simulink model "New_model"  (R2021a)
settings: Solver=ode14x  StartTime=0.0  StopTime=100  FixedStep=0.1  RelTol=1e-3
undefined symbols (not defined in the file or in its folder): Ion, Lithium
libraries: fl_lib x29, spsBatteryLib x26, nesl_utility x14, ee_lib x4, sdl_lib x3, spsSeriesRLCLoadLib x2, spsVoltageMeasurementLib x2, spspowerguiLib x2
settings Model: Creator=Zhi Hang  LastModifiedBy=msipc

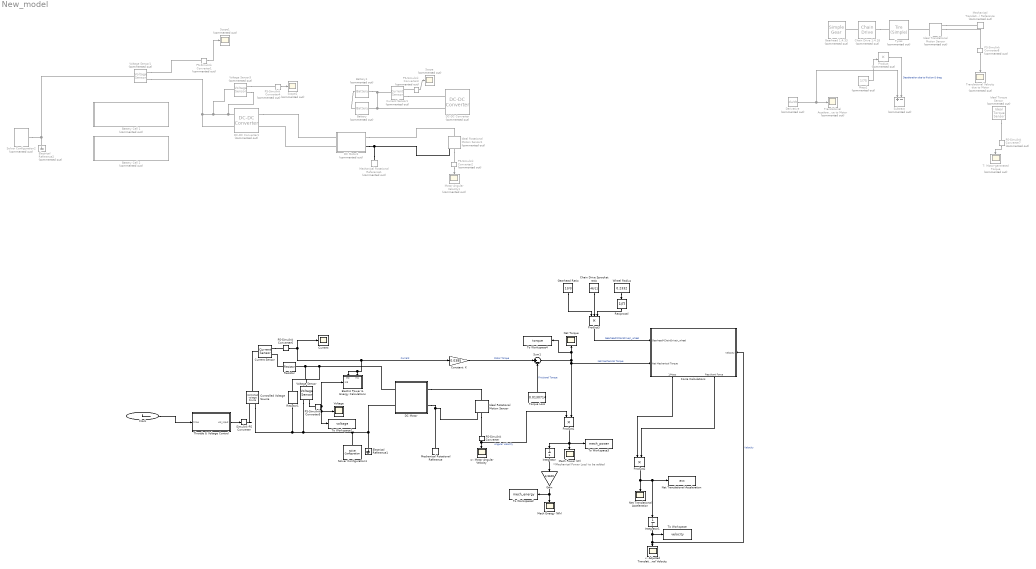
== system New_model ==
  note: *(Mechanical Power Loss) to be added
  Battery : ee_lib/Sources/Battery  Commented=on  Vnom=52 V  prm_dir=1  R1_dis=2 Ohm  R1_ch=2 Ohm  R1=0.26 Ohm  prm_AH=2  AH=2.95 hr*A  V1=45.5 V  AH1=1.385 hr*A  prm_R2=1  R2=2000 Ohm  prm_dyn=1  Rp1=0.005 Ohm  tau1=30 s  Rp2=0.005 Ohm  tau2=30 s  Rp3=0.005 Ohm  tau3=30 s  Rp4=0.005 Ohm  tau4=30 s  Rp5=0.005 Ohm  tau5=30 s  prm_fade=1  N_fade=100  AH_fade=45 hr*A  R1_fade=2.02 Ohm  R1_ch_fade=2.02 Ohm  V1_fade=10.35 V  prm_age=1  prm_age_OCV=1  OCV_age=0.9  SOC_age=60  Tmeas_age=298.15 K  delta_time_age_vec=[0] d  temperature_age_vec=[273] K  OCV_scaling_age=2.2134e6  OCV_offset_age=1.632e6  temp_exp_age=0.515833569 V  t_exp_age=0.75  i_specify=off  i_priority=None  i=0 A  i_nominal_specify=off  i_nominal_unit=A  i_nominal_value=1  v_specify=off  v_priority=None  v=0 V  v_nominal_specify=off  v_nominal_unit=V  v_nominal_value=1  charge_specify=on  charge_priority=High  charge=2.95 hr*A  charge_nominal_specify=off  charge_nominal_unit=hr*A  charge_nominal_value=1  num_cycles_specify=off  num_cycles_priority=High  num_cycles=0  num_cycles_nominal_specify=off  num_cycles_nominal_unit=1  num_cycles_nominal_value=1  thermal_mass=30000 J/K  Tmeas=298.15 K  Vnom_T2=12 V  R1_T2=2.2 Ohm  R1_T2_dis=2.2 Ohm  R1_T2_ch=2.2 Ohm  V1_T2=11.4 V  R2_T2=2200 Ohm  Rp1_T2=0.005 Ohm  tau1_T2=30 s  Rp2_T2=0.005 Ohm  tau2_T2=30 s  Rp3_T2=0.005 Ohm  tau3_T2=30 s  Rp4_T2=0.005 Ohm  tau4_T2=30 s  Rp5_T2=0.005 Ohm  tau5_T2=30 s  Tmeas2=273.15 K  temperature_specify=off  temperature_priority=High  temperature=298.15 K  temperature_nominal_specify=off  temperature_nominal_unit=K  temperature_nominal_value=1
  Battery Cell 1 : Subsystem  Commented=on
  Battery Cell 2 : Subsystem  Commented=on
  Battery1 : ee_lib/Sources/Battery  Commented=on  Vnom=52 V  prm_dir=1  R1_dis=2 Ohm  R1_ch=2 Ohm  R1=0.26 Ohm  prm_AH=2  AH=2.95 hr*A  V1=45.5 V  AH1=1.385 hr*A  prm_R2=1  R2=2000 Ohm  prm_dyn=1  Rp1=0.005 Ohm  tau1=30 s  Rp2=0.005 Ohm  tau2=30 s  Rp3=0.005 Ohm  tau3=30 s  Rp4=0.005 Ohm  tau4=30 s  Rp5=0.005 Ohm  tau5=30 s  prm_fade=1  N_fade=100  AH_fade=45 hr*A  R1_fade=2.02 Ohm  R1_ch_fade=2.02 Ohm  V1_fade=10.35 V  prm_age=1  prm_age_OCV=1  OCV_age=0.9  SOC_age=60  Tmeas_age=298.15 K  delta_time_age_vec=[0] d  temperature_age_vec=[273] K  OCV_scaling_age=2.2134e6  OCV_offset_age=1.632e6  temp_exp_age=0.515833569 V  t_exp_age=0.75  i_specify=off  i_priority=None  i=0 A  i_nominal_specify=off  i_nominal_unit=A  i_nominal_value=1  v_specify=off  v_priority=None  v=0 V  v_nominal_specify=off  v_nominal_unit=V  v_nominal_value=1  charge_specify=on  charge_priority=High  charge=2.95 hr*A  charge_nominal_specify=off  charge_nominal_unit=hr*A  charge_nominal_value=1  num_cycles_specify=off  num_cycles_priority=High  num_cycles=0  num_cycles_nominal_specify=off  num_cycles_nominal_unit=1  num_cycles_nominal_value=1  thermal_mass=30000 J/K  Tmeas=298.15 K  Vnom_T2=12 V  R1_T2=2.2 Ohm  R1_T2_dis=2.2 Ohm  R1_T2_ch=2.2 Ohm  V1_T2=11.4 V  R2_T2=2200 Ohm  Rp1_T2=0.005 Ohm  tau1_T2=30 s  Rp2_T2=0.005 Ohm  tau2_T2=30 s  Rp3_T2=0.005 Ohm  tau3_T2=30 s  Rp4_T2=0.005 Ohm  tau4_T2=30 s  Rp5_T2=0.005 Ohm  tau5_T2=30 s  Tmeas2=273.15 K  temperature_specify=off  temperature_priority=High  temperature=298.15 K  temperature_nominal_specify=off  temperature_nominal_unit=K  temperature_nominal_value=1
  Chain Drive 1:4.18 : sdl_lib/Couplings & Drives/Chain Drive  Commented=on  chain_model=sdl.enum.chain_model.ideal  radius_a=20 mm  radius_b=20*46/11 mm  slack=50 mm  k_chain=1e5 N/m  mu_visc_chain=5 N/(m/s)  mu_visc_a=0 N*m/(rad/s)  mu_visc_b=0 N*m/(rad/s)  breakable=sdl.enum.max_tension.off  F_max=1e6 N  x_specify=off  x_priority=High  x=0 mm  x_nominal_specify=off  x_nominal_unit=mm  x_nominal_value=1
      settings: SourceProductBaseCode=LD  InternalSimscapePortConfiguration="{\"Bottom\":[],\"Left\":[{\"id\":\"A\",\"label\":\"A\",\"type\":\"foundation.mechanical.rotational.rotational\"}],\"Right\":[{\"id\":\"B\",\"label\":\"B\",\"type\":\"foundation.mechanical.rotational.rotational\"}],\"Top\":[]}"
  Chain Drive Sprocket ratio : Constant  Value=46/11
  Clock : Clock
  Constant: K : Gain  Gain=0.0385
  Controlled Voltage Source : fl_lib/Electrical/Electrical Sources/Controlled Voltage Source
  Current : Scope
  Current Sensor : fl_lib/Electrical/Electrical Sensors/Current Sensor
  Current Sensor1 : fl_lib/Electrical/Electrical Sensors/Current Sensor  Commented=on
  DC Motor : Subsystem
  DC Motor1 : Subsystem  Commented=on
  DC-DC Converter : ee_lib/Semiconductors & Converters/Converters/DC-DC Converter  Commented=on  Vref_option=ee.enum.converters.voltageref.internal  v_ref=12 V  P_rated=40 W  droop_param=ee.enum.converters.droop.value  reversible=ee.enum.converters.directionality.unidirectional  losses_option=ee.enum.converters.lossesOption.proportionalToSquaredCurrent  P_fixed=1 W  model_dynamics=ee.enum.converters.dynamics.no  i1_max=15 A  enable_fault=ee.enum.faults.faultEnable.no  fault_condition=ee.enum.faults.faultInputCondition.greaterThan  fault_threshold=0.5  droop=0.8 V/A  droop_percent=2  tau=0.02 s  v_ini=10 V  G_diode=1e-8 1/Ohm  eff_rated=80  i_eff_vec=[1, 2, 3, 4] A  eff_vec=[90, 80, 70, 60]  thermal_mass=100 J/K  initial_temperature=298.15 K  T_eff_vec=[280, 300, 320] K  eff_2D_table=[90, 85, 80; 80, 75, 70; 70, 65, 60; 60, 55, 50]
      settings: SourceProductBaseCode=PS  InternalSimscapePortConfiguration="{\"Bottom\":[],\"Left\":[{\"id\":\"p1\",\"label\":\"1+\",\"type\":\"foundation.electrical.electrical\"},{\"id\":\"n1\",\"label\":\"1-\",\"type\":\"foundation.electrical.electrical\"}],\"Right\":[{\"id\":\"p2\",\"label\":\"2+\",\"type\":\"foundation.electrical.electrical\"},{\"id\":\"n2\",\"label\":\"2-\",\"type\":\"foundation.electrical.electrical\"}],\"Top\":[]}"
  DC-DC Converter1 : ee_lib/Semiconductors & Converters/Converters/DC-DC Converter  Commented=on  Vref_option=ee.enum.converters.voltageref.internal  v_ref=12 V  P_rated=40 W  droop_param=ee.enum.converters.droop.value  reversible=ee.enum.converters.directionality.unidirectional  losses_option=ee.enum.converters.lossesOption.proportionalToSquaredCurrent  P_fixed=1 W  model_dynamics=ee.enum.converters.dynamics.no  i1_max=15 A  enable_fault=ee.enum.faults.faultEnable.no  fault_condition=ee.enum.faults.faultInputCondition.greaterThan  fault_threshold=0.5  droop=0.8 V/A  droop_percent=2  tau=0.02 s  v_ini=10 V  G_diode=1e-8 1/Ohm  eff_rated=91  i_eff_vec=[1, 2, 3, 4] A  eff_vec=[90, 80, 70, 60]  thermal_mass=100 J/K  initial_temperature=298.15 K  T_eff_vec=[280, 300, 320] K  eff_2D_table=[90, 85, 80; 80, 75, 70; 70, 65, 60; 60, 55, 50]
      settings: SourceProductBaseCode=PS  InternalSimscapePortConfiguration="{\"Bottom\":[],\"Left\":[{\"id\":\"p1\",\"label\":\"1+\",\"type\":\"foundation.electrical.electrical\"},{\"id\":\"n1\",\"label\":\"1-\",\"type\":\"foundation.electrical.electrical\"}],\"Right\":[{\"id\":\"p2\",\"label\":\"2+\",\"type\":\"foundation.electrical.electrical\"},{\"id\":\"n2\",\"label\":\"2-\",\"type\":\"foundation.electrical.electrical\"}],\"Top\":[]}"
  Derivative : Derivative  Commented=on
  Electric Power & Energy Calculations : Subsystem
      settings: PortSchema="{\"entries\":[{\"content\":{\"sides\":[{\"content\":{\"connectorIds\":[\"In1\",\"In2\"]},\"type\":\"ConnectorPlacement.EquallySpacedRectSide\",\"uuid\":\"82b9f0de-574e-4e17-acb9-bed6a2542387\"},{\"content\":{\"connectorIds\":[],\"side\":\"RIGHT\"},\"type\":\"ConnectorPlacement.EquallySpacedRectSide\",\"uuid\":\"9cdc9c20-443d-4f74-aa57-a6f03633b23a\"},{\"content\":{\"connectorIds\":[],\"side\":\"TOP\"},\"type\":\"ConnectorPlacement.EquallySpacedRectSide\",\"uuid\":\"5887af2a-3520-4210-9b68-9038b3c81c3d\"},{\"content\":{\"connectorIds\":[\"In3\"],\"side\":\"BOTTOM\"},\"type\":\"ConnectorPlacement.EquallySpacedRectSide\",\"uuid\":\"9e0946f9-9655-43ed-bd46-b30a5293a4ce\"}]},\"type\":\"ConnectorPlacement.EquallySpacedConnector\",\"uuid\":\"9fe55d6d-7bcf-4897-9064-2d765cec3f3f\"}],\"packageUris\":[\"http://schema.mathworks.com/mf0/Connector/R2020b\"],\"version\":\"1.0\"}"
  Electrical Reference1 : fl_lib/Electrical/Electrical Elements/Electrical Reference
  Electrical Reference2 : fl_lib/Electrical/Electrical Elements/Electrical Reference  Commented=on
  Force Calculations : Subsystem
      settings: PortSchema="{\"entries\":[{\"content\":{\"sides\":[{\"content\":{\"connectorIds\":[\"In1\",\"In2\"]},\"type\":\"ConnectorPlacement.EquallySpacedRectSide\",\"uuid\":\"cc3dc385-e02b-45e3-b13c-6583fb37f4e9\"},{\"content\":{\"connectorIds\":[\"In3\"],\"side\":\"RIGHT\"},\"type\":\"ConnectorPlacement.EquallySpacedRectSide\",\"uuid\":\"d2c64c73-4662-4205-87fa-010500d01f5e\"},{\"content\":{\"connectorIds\":[],\"side\":\"TOP\"},\"type\":\"ConnectorPlacement.EquallySpacedRectSide\",\"uuid\":\"e476453e-7c1d-4526-b790-afcebe39b1ff\"},{\"content\":{\"connectorIds\":[\"Out1\",\"Out2\"],\"side\":\"BOTTOM\"},\"type\":\"ConnectorPlacement.EquallySpacedRectSide\",\"uuid\":\"93b3e609-0036-4bd4-a5db-553470fdefa2\"}]},\"type\":\"ConnectorPlacement.EquallySpacedConnector\",\"uuid\":\"e3829ec2-f118-48d6-87d1-cf59a67f9f8c\"}],\"packageUris\":[\"http://schema.mathworks.com/mf0/Connector/R2020b\"],\"version\":\"1.0\"}"
  Gain : Gain  Gain=1/3600
  Gearhead 1:4.33 : sdl_lib/Gears/Simple Gear  Commented=on  ratio=4.33  rotation_direction=sdl.enum.shaftOutputDirection.same  friction_model=sdl.enum.gear_efficiencies_load.constant  mu_visc=[0, 0] N*m/(rad/s)  T_noload=0.1 N*m  T_nom=5 N*m  efficiency_nom=0.8  efficiency=0.9  temperature_TLU=[280, 300, 320] K  load_TLU=[1, 5, 10] N*m  efficiency_TLU=[.95, .9, .85]  efficiency_TLU2=[.85, .8, .75; .95, .9, .85; .85, .8, .7]  w_thr=0.01 rad/s  pwr_thr=0.001 W  thermal_mass=50 J/K  enable_faults=simscape.enum.onoff.off  efficiency_fault=0.05  external_fault=simscape.enum.onoff.off  temporal_fault=simscape.enum.onoff.off  fault_time=5 s  fault_angles=pi / 12 rad  report_fault=simscape.enum.assert.action.none  temperature_specify=off  temperature_priority=High  temperature=300 K  temperature_nominal_specify=off  temperature_nominal_unit=K  temperature_nominal_value=1
  Gearhead Ratio : Constant  Value=13/3
  Ideal Rotational Motion Sensor : fl_lib/Mechanical/Mechanical Sensors/Ideal Rotational Motion Sensor  wrap_angle=simscape.enum.onoff.off  offset=0 rad
  Ideal Rotational Motion Sensor1 : fl_lib/Mechanical/Mechanical Sensors/Ideal Rotational Motion Sensor  Commented=on  wrap_angle=simscape.enum.onoff.off  offset=0 rad
  Ideal Torque Sensor : fl_lib/Mechanical/Mechanical Sensors/Ideal Torque Sensor  Commented=on
  Ideal Translational Motion Sensor : fl_lib/Mechanical/Mechanical Sensors/Ideal Translational Motion Sensor  Commented=on  offset=0 m
  Integrator : Integrator
  Integrator1 : Integrator
  Mass1 : Constant  Commented=on  Value=1/75
  Mech Energy (Wh) : Scope
  Mech Power (W) : Scope
  Mechanical Rotational Reference : fl_lib/Mechanical/Rotational Elements/Mechanical Rotational Reference
  Mechanical Rotational Reference1 : fl_lib/Mechanical/Rotational Elements/Mechanical Rotational Reference  Commented=on
  Mechanical Translational Reference : fl_lib/Mechanical/Translational Elements/Mechanical Translational Reference  Commented=on
  Motor Angular Velocity1 : Scope  Commented=on
  Net Torque : Scope
  Net Translational Acceleration : Scope
  Net Translational Acceleration : ToWorkspace  VariableName=acc  SaveFormat=Timeseries  SampleTime=-1
  PS-Simulink Converter : nesl_utility/PS-Simulink Converter  PhysicalDomain=network_engine_domain  SubClassName=ps_output  LeftPortType=input  RightPortType=output  PseudoPeriodic=off  Frequencies=[]  Unit=inherit  AffineConversion=off
      settings: SourceProductBaseCode=PW,SS
  PS-Simulink Converter{1..4,7..8} (6 alike) : nesl_utility/PS-Simulink Converter  Commented=on  PhysicalDomain=network_engine_domain  SubClassName=ps_output  LeftPortType=input  RightPortType=output  PseudoPeriodic=off  Frequencies=[]  Unit=inherit  AffineConversion=off
      settings: SourceProductBaseCode=PW,SS
  PS-Simulink Converter5 : nesl_utility/PS-Simulink Converter  PhysicalDomain=network_engine_domain  SubClassName=ps_output  LeftPortType=input  RightPortType=output  PseudoPeriodic=off  Frequencies=[]  Unit=inherit  AffineConversion=off
      settings: SourceProductBaseCode=PW,SS
  PS-Simulink Converter6 : nesl_utility/PS-Simulink Converter  PhysicalDomain=network_engine_domain  SubClassName=ps_output  LeftPortType=input  RightPortType=output  PseudoPeriodic=off  Frequencies=[]  Unit=inherit  AffineConversion=off
      settings: SourceProductBaseCode=PW,SS
  Product : Product  Commented=on
  Product1 : Product
  Product2 : Product
  Product3 : Product  Inputs=3
  Reciprocal : Product  Inputs=/
  Resistor : fl_lib/Electrical/Electrical Elements/Resistor  R=1 Ohm  i_specify=off  i_priority=None  i=0 A  i_nominal_specify=off  i_nominal_unit=A  i_nominal_value=1  v_specify=off  v_priority=None  v=0 V  v_nominal_specify=off  v_nominal_unit=V  v_nominal_value=1
  Resistor1 : fl_lib/Electrical/Electrical Elements/Resistor  R=30 Ohm  i_specify=off  i_priority=None  i=0 A  i_nominal_specify=off  i_nominal_unit=A  i_nominal_value=1  v_specify=off  v_priority=None  v=0 V  v_nominal_specify=off  v_nominal_unit=V  v_nominal_value=1
  Scope : Scope  Commented=on
  Scope1 : Scope  Commented=on
  Scope2 : Scope  Commented=on
  Simulink-PS Converter : nesl_utility/Simulink-PS Converter  PhysicalDomain=network_engine_domain  SubClassName=ps_input  LeftPortType=input  RightPortType=output  PseudoPeriodic=off  Frequencies=[]  NoiseDistribution=none  NoiseParameters=[]  Unit=1  AffineConversion=off  FilteringAndDerivatives=filter  SimscapeFilterOrder=1  InputFilterTimeConstant=0.001  UdotUserProvided=0
      settings: SourceProductBaseCode=PW,SS
  Solver Configuration1 : nesl_utility/Solver Configuration  PhysicalDomain=network_engine_domain  SubClassName=solver  LeftPortType=input  RightPortType=generic  Tones=[]  Harmonics=[]  SimulateNoise=off  Profile=off  UseLocalSampling=off  EnableSwitchedLinearOptims=on  FrequencyDomain=off  UseCCode=off  RelTol=0.001  AbsTol=1e-06  MinStep=1e-09  ToWorkspace=off  RevertToSquareIcSolve=off  NumHomotopyIterations=100  PhasorMode=off  PhasorModeNumHarmonics=1  DoDC=off  ResidualTolerance=1e-09  UseLocalSolver=off  LocalSolverChoice=NE_BACKWARD_EULER_ADVANCER  LocalSolverSampleTime=0.001  DoFixedCost=off  MaxNonlinIter=3  MaxModeIter=2  ComputeImpulses=off  ImpulseIterations=2  LinearAlgebra=auto  EquationFormulation=NE_TIME_EF  DelaysMemoryBudget=1024  AutomaticFiltering=on  FilteringTimeConstant=0.001  PartitionStorageMethod=AS_NEEDED  PartitionMemoryBudget=1024  PartitionMethod=ROBUST
      settings: SourceProductBaseCode=PW,SS
  Solver Configuration2 : nesl_utility/Solver Configuration  Commented=on  PhysicalDomain=network_engine_domain  SubClassName=solver  LeftPortType=input  RightPortType=generic  Tones=[]  Harmonics=[]  SimulateNoise=off  Profile=off  UseLocalSampling=off  EnableSwitchedLinearOptims=on  FrequencyDomain=off  UseCCode=off  RelTol=0.001  AbsTol=1e-06  MinStep=1e-09  ToWorkspace=off  RevertToSquareIcSolve=off  NumHomotopyIterations=100  PhasorMode=off  PhasorModeNumHarmonics=1  DoDC=off  ResidualTolerance=1e-09  UseLocalSolver=off  LocalSolverChoice=NE_BACKWARD_EULER_ADVANCER  LocalSolverSampleTime=0.001  DoFixedCost=off  MaxNonlinIter=3  MaxModeIter=2  ComputeImpulses=off  ImpulseIterations=2  LinearAlgebra=auto  EquationFormulation=NE_TIME_EF  DelaysMemoryBudget=1024  AutomaticFiltering=on  FilteringTimeConstant=0.001  PartitionStorageMethod=AS_NEEDED  PartitionMemoryBudget=1024  PartitionMethod=ROBUST
      settings: SourceProductBaseCode=PW,SS
  Subtract : Sum  Commented=on  Inputs=+-
  Sum1 : Sum  Inputs=|+-
  T: Motor-generated Torque : Scope  Commented=on
  Throttle & Voltage Control : MATLAB Function  TreatAsAtomicUnit=on
  To Workspace : ToWorkspace  VariableName=velocity  SaveFormat=Timeseries  SampleTime=-1
  To Workspace1 : ToWorkspace  VariableName=voltage  SaveFormat=Timeseries  SampleTime=-1
  To Workspace2 : ToWorkspace  VariableName=mech_energy  SaveFormat=Timeseries  SampleTime=-1
  To Workspace3 : ToWorkspace  VariableName=mech_power  SaveFormat=Timeseries  SampleTime=-1
  To Workspace4 : ToWorkspace  VariableName=torque  SaveFormat=Timeseries  SampleTime=-1
  Torque Loss : Constant  Value=0.0130714
  Translational Acceleration due to Motor : Scope  Commented=on
  Translational Velocity due to Motor : Scope  Commented=on
  Tyres : sdl_lib/Tires & Vehicles/Tire (Simple)  Commented=on  r_tire=0.2332 m  model_compliance=0  stiffness=1e6 N/m  damping=1000 N/(m/s)  model_inertia=0  tire_inertia=0.5 kg*m^2  initial_velocity=0 rad/s
      settings: SourceProductBaseCode=LD  InternalSimscapePortConfiguration="{\"Bottom\":[],\"Left\":[{\"id\":\"A\",\"label\":\"A\",\"type\":\"foundation.mechanical.rotational.rotational\"}],\"Right\":[{\"id\":\"H\",\"label\":\"H\",\"type\":\"foundation.mechanical.translational.translational\"}],\"Top\":[]}"
  Voltage : Scope
  Voltage Sensor : fl_lib/Electrical/Electrical Sensors/Voltage Sensor
  Voltage Sensor1 : fl_lib/Electrical/Electrical Sensors/Voltage Sensor  Commented=on
  Voltage Sensor3 : fl_lib/Electrical/Electrical Sensors/Voltage Sensor  Commented=on
  Wheel Radius : Constant  Value=0.2332
  v: Adjusted Translational Velocity : Scope
  w: Motor Angular Velocity : Scope
  wires:
  PS-Simulink Converter/1 -> Product1/1, w: Motor Angular Velocity/1  "Angular Velocity"
  PS-Simulink Converter3/1 -> Scope/1
  PS-Simulink Converter1/1 -> Scope1/1
  PS-Simulink Converter2/1 -> Motor Angular Velocity1/1
  PS-Simulink Converter4/1 -> Scope2/1
  PS-Simulink Converter8/1 -> Translational Velocity due to Motor/1
  Derivative/1 -> Subtract/1, Translational Acceleration due to Motor/1
  Mass1/1 -> Product/2
  Clock/1 -> Throttle & Voltage Control/1(time)
  Product/1 -> Subtract/2  "Deceleration due to friction & drag"
  Throttle & Voltage Control/1(vol_input) -> Simulink-PS Converter/1
  Constant: K/1 -> Sum1/1  "Motor Torque"
  PS-Simulink Converter6/1 -> Constant: K/1, Electric Power & Energy Calculations/2(In2), Electric Power & Energy Calculations/1(In1), Current/1  "Current"
  PS-Simulink Converter5/1 -> To Workspace1/1, Voltage/1, Electric Power & Energy Calculations/3(In3)
  PS-Simulink Converter7/1 -> T: Motor-generated Torque/1
  Product2/1 -> Net Translational Acceleration/1, Integrator1/1, Net Translational Acceleration/1
  Integrator1/1 -> v: Adjusted Translational Velocity/1, Force Calculations/3(Velocity), To Workspace/1  "Velocity"
  Sum1/1 -> Product1/2, Force Calculations/2(Net Mechanical Torque), Net Torque/1, To Workspace4/1  "Net Mechanical Torque"
  Torque Loss/1 -> Sum1/2  "Frictional Torque"
  Product1/1 -> Mech Power (W)/1, To Workspace3/1, Integrator/1
  Integrator/1 -> Gain/1
  Wheel Radius/1 -> Reciprocal/1
  Gearhead Ratio/1 -> Product3/1
  Chain Drive Sprocket ratio/1 -> Product3/2
  Reciprocal/1 -> Product3/3
  Gain/1 -> Mech Energy (Wh)/1, To Workspace2/1
  Product3/1 -> Force Calculations/1(Gearhead*ChainDrive/r_wheel)  "Gearhead*ChainDrive/r_wheel"
  Force Calculations/1(1/Mass) -> Product2/1
  Force Calculations/2(Resultant Force) -> Product2/2
  connections:
  DC Motor/RConn1 -- Ideal Rotational Motion Sensor/LConn1
  DC Motor/RConn2 -- Ideal Rotational Motion Sensor/RConn1 -- Mechanical Rotational Reference/LConn1
  Ideal Rotational Motion Sensor/RConn2 -- PS-Simulink Converter/LConn1
  Battery1/RConn1 -- Current Sensor1/LConn1 -- DC-DC Converter/LConn2 -- Battery/RConn1
  Battery/LConn1 -- Battery1/LConn1
  DC Motor/LConn2 -- Controlled Voltage Source/RConn2 -- Resistor1/RConn1 -- Voltage Sensor/RConn2 -- Solver Configuration1/RConn1 -- Electrical Reference1/LConn1
  Current Sensor1/RConn2 -- DC-DC Converter/LConn1
  PS-Simulink Converter3/LConn1 -- Current Sensor1/RConn1
  Solver Configuration2/RConn1 -- Electrical Reference2/LConn1 -- Voltage Sensor1/LConn1
  Voltage Sensor1/RConn1 -- PS-Simulink Converter1/LConn1
  Mechanical Rotational Reference1/LConn1 -- Ideal Rotational Motion Sensor1/RConn1 -- DC Motor1/RConn2
  DC Motor1/RConn1 -- Ideal Rotational Motion Sensor1/LConn1
  Ideal Rotational Motion Sensor1/RConn2 -- PS-Simulink Converter2/LConn1
  DC-DC Converter1/RConn1 -- DC Motor1/LConn1
  DC Motor1/LConn2 -- DC-DC Converter1/RConn2
  Voltage Sensor1/RConn2 -- Voltage Sensor3/LConn1 -- Voltage Sensor3/RConn2 -- DC-DC Converter1/LConn1 -- DC-DC Converter1/LConn2
  Voltage Sensor3/RConn1 -- PS-Simulink Converter4/LConn1
  Chain Drive 1:4.18/LConn1 -- Gearhead 1:4.33/RConn1
  Voltage Sensor/RConn1 -- PS-Simulink Converter5/LConn1
  Chain Drive 1:4.18/RConn1 -- Tyres/LConn1
  Ideal Translational Motion Sensor/LConn1 -- Tyres/RConn1
  Ideal Translational Motion Sensor/RConn1 -- Mechanical Translational Reference/LConn1
  Ideal Translational Motion Sensor/RConn2 -- PS-Simulink Converter8/LConn1
  Simulink-PS Converter/RConn1 -- Controlled Voltage Source/RConn1
  DC Motor/LConn1 -- Voltage Sensor/LConn1 -- Resistor1/LConn1 -- Resistor/RConn1
  Current Sensor/RConn1 -- PS-Simulink Converter6/LConn1
  Ideal Torque Sensor/RConn2 -- PS-Simulink Converter7/LConn1
  Current Sensor/LConn1 -- Controlled Voltage Source/LConn1
  Resistor/LConn1 -- Current Sensor/RConn2

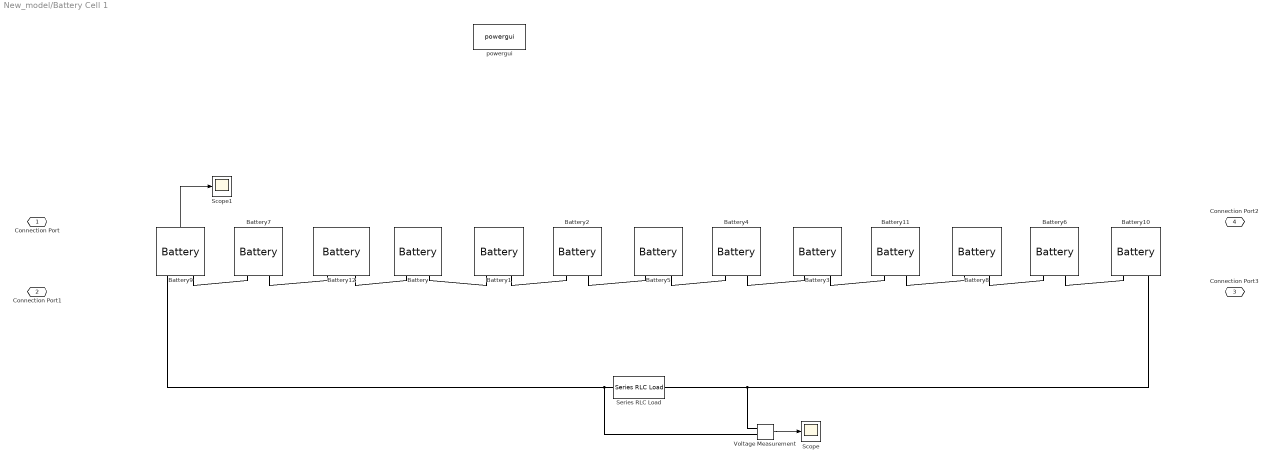
== system New_model/Battery Cell 1 ==
  Battery{,1..12} (13 alike) : spsBatteryLib/Battery  BatType=Lithium-Ion  ShowTempParam=off  ThermalPreset=no  ShowAgeParam=off  NomV=3.61  NomQ=2.95  SOC=100  Batt_Tr=1  PresetModel=off  MaxQ=2.95  MinV=2.5  FullV=4.1  Dis_rate=5  R=0.03  Normal_OP=1.65  expZone=[3.95 0.1]  current=[0 1 2 3 4 5]  Units=Time  Tci=20  NomT=20  T2=-30  MaxQ2=4.8  FullV2=7.1  Normal_OP2=5.655  expZone2="[6.58           1]"  Rca=0.6  ti=2000  Dp=0  Neq0=0  Tsim=1e6  Ta1=25  Qeol=5.4*0.9  Reol=0.013333*1.2  Char_age=[2.3478, 3]  Dis_age=[2.3478, 10]  N1=1500  N2=10500  N3=1000  N4=1400  Ta2=45  N5=950
  Scope : Scope
  Scope1 : Scope
  Series RLC Load : spsSeriesRLCLoadLib/Series RLC Load  LConnTagsString=a  RConnTagsString=__new0  NominalVoltage=1000  NominalFrequency=60  ActivePower=10e4  InductivePower=0  CapacitivePower=0  Setx0=off  InitialVoltage=0  SetiL0=off  InitialCurrent=0  Measurements=None  LoadType=constant Z
  Voltage Measurement : spsVoltageMeasurementLib/Voltage Measurement  PhasorSimulation=off  OutputType=Complex  PSBequivalent=0
  powergui : spspowerguiLib/powergui  Priority=1  SimulationMode=Continuous  SampleTime=50e-6  frequency=60  Iterations=50  frequencyindice=0  Pbase=100e6  ErrMax=1e-4  UnitsV=kV  UnitsW=MW  buscounter=0  FunctionMessages=off  echomessages=off  EnableUseOfTLC=off  CurrentSourceSwitches=off  DisableSnubberDevices=off  DisableRonSwitches=off  DisableVfSwitches=off  DisplayEquations=off  AutomaticDiscreteSolvers=off  SolverType=Tustin/Backward Euler (TBE)  Interpol=off  ExternalGateDelay=off  methode=off  Ts=100  x0status=blocks  SPID=on  SwTol=0  HookPort=off  NonlinearTolerance=1e-4  nMaxIteration=100  ContinueOnMaxIteration=off  RestoreLinks=warning  ResistiveCurrentMeasurement=off  Frange=[0:2:500]  Ylog=off  Xlog=on  ShowGrid=off  save=off  variable=ZData  structure=0  ZoomFFT=off  StartTime=0.0  cycles=1  DisplayStyle=1  fundamental=60  FreqAxis=off  MaxFrequency=1000  frequencyindicesteady=1  RmsSteady=1  display=off
  Connection Port : PMIOPort  Side=Left
  Connection Port1 : PMIOPort  Port=2  Side=Left
  Connection Port3 : PMIOPort  Port=3  Side=Right
  Connection Port2 : PMIOPort  Port=4  Side=Right
  wires:
  Voltage Measurement/1 -> Scope/1
  Battery9/1 -> Scope1/1
  connections:
  Battery9/LConn1 -- Battery7/LConn2
  Battery7/LConn1 -- Battery12/LConn2
  Battery12/LConn1 -- Battery/LConn2
  Battery1/LConn2 -- Battery/LConn1
  Battery1/LConn1 -- Battery2/LConn2
  Battery2/LConn1 -- Battery5/LConn2
  Battery5/LConn1 -- Battery4/LConn2
  Battery4/LConn1 -- Battery3/LConn2
  Battery3/LConn1 -- Battery11/LConn2
  Battery11/LConn1 -- Battery8/LConn2
  Battery8/LConn1 -- Battery6/LConn2
  Battery6/LConn1 -- Battery10/LConn2
  Battery9/LConn2 -- Voltage Measurement/LConn2 -- Series RLC Load/LConn1
  Battery10/LConn1 -- Voltage Measurement/LConn1 -- Series RLC Load/RConn1

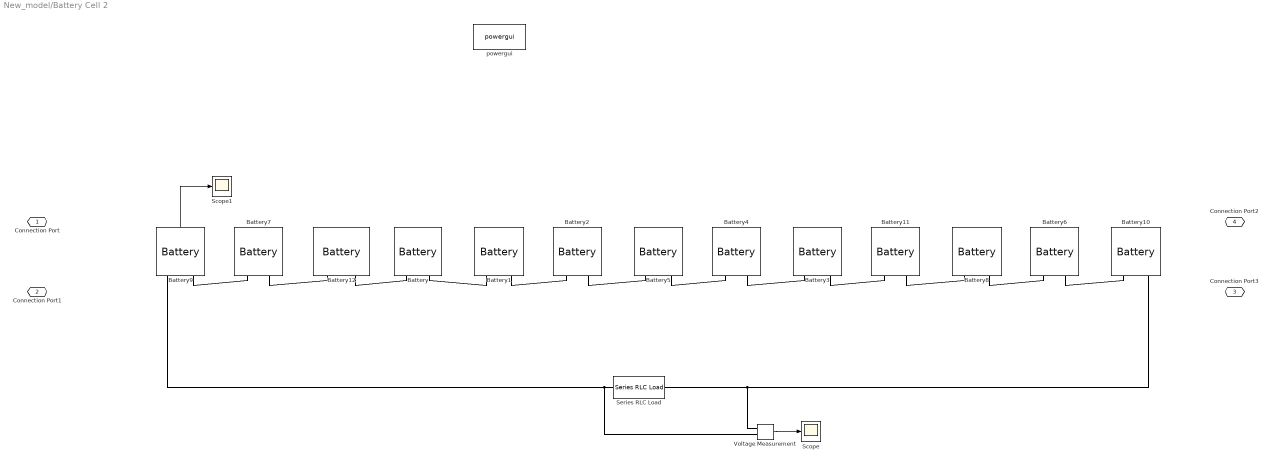
== system New_model/Battery Cell 2 ==
  Battery{,1..12} (13 alike) : spsBatteryLib/Battery  BatType=Lithium-Ion  ShowTempParam=off  ThermalPreset=no  ShowAgeParam=off  NomV=3.61  NomQ=2.95  SOC=100  Batt_Tr=1  PresetModel=off  MaxQ=2.95  MinV=2.5  FullV=4.1  Dis_rate=5  R=0.03  Normal_OP=1.65  expZone=[3.95 0.1]  current=[0 1 2 3 4 5]  Units=Time  Tci=20  NomT=20  T2=-30  MaxQ2=4.8  FullV2=7.1  Normal_OP2=5.655  expZone2="[6.58           1]"  Rca=0.6  ti=2000  Dp=0  Neq0=0  Tsim=1e6  Ta1=25  Qeol=5.4*0.9  Reol=0.013333*1.2  Char_age=[2.3478, 3]  Dis_age=[2.3478, 10]  N1=1500  N2=10500  N3=1000  N4=1400  Ta2=45  N5=950
  Scope : Scope
  Scope1 : Scope
  Series RLC Load : spsSeriesRLCLoadLib/Series RLC Load  LConnTagsString=a  RConnTagsString=__new0  NominalVoltage=1000  NominalFrequency=60  ActivePower=10e4  InductivePower=0  CapacitivePower=0  Setx0=off  InitialVoltage=0  SetiL0=off  InitialCurrent=0  Measurements=None  LoadType=constant Z
  Voltage Measurement : spsVoltageMeasurementLib/Voltage Measurement  PhasorSimulation=off  OutputType=Complex  PSBequivalent=0
  powergui : spspowerguiLib/powergui  Priority=1  SimulationMode=Continuous  SampleTime=50e-6  frequency=60  Iterations=50  frequencyindice=0  Pbase=100e6  ErrMax=1e-4  UnitsV=kV  UnitsW=MW  buscounter=0  FunctionMessages=off  echomessages=off  EnableUseOfTLC=off  CurrentSourceSwitches=off  DisableSnubberDevices=off  DisableRonSwitches=off  DisableVfSwitches=off  DisplayEquations=off  AutomaticDiscreteSolvers=off  SolverType=Tustin/Backward Euler (TBE)  Interpol=off  ExternalGateDelay=off  methode=off  Ts=100  x0status=blocks  SPID=on  SwTol=0  HookPort=off  NonlinearTolerance=1e-4  nMaxIteration=100  ContinueOnMaxIteration=off  RestoreLinks=warning  ResistiveCurrentMeasurement=off  Frange=[0:2:500]  Ylog=off  Xlog=on  ShowGrid=off  save=off  variable=ZData  structure=0  ZoomFFT=off  StartTime=0.0  cycles=1  DisplayStyle=1  fundamental=60  FreqAxis=off  MaxFrequency=1000  frequencyindicesteady=1  RmsSteady=1  display=off
  Connection Port : PMIOPort  Side=Left
  Connection Port1 : PMIOPort  Port=2  Side=Left
  Connection Port3 : PMIOPort  Port=3  Side=Right
  Connection Port2 : PMIOPort  Port=4  Side=Right
  wires:
  Voltage Measurement/1 -> Scope/1
  Battery9/1 -> Scope1/1
  connections:
  Battery9/LConn1 -- Battery7/LConn2
  Battery7/LConn1 -- Battery12/LConn2
  Battery12/LConn1 -- Battery/LConn2
  Battery1/LConn2 -- Battery/LConn1
  Battery1/LConn1 -- Battery2/LConn2
  Battery2/LConn1 -- Battery5/LConn2
  Battery5/LConn1 -- Battery4/LConn2
  Battery4/LConn1 -- Battery3/LConn2
  Battery3/LConn1 -- Battery11/LConn2
  Battery11/LConn1 -- Battery8/LConn2
  Battery8/LConn1 -- Battery6/LConn2
  Battery6/LConn1 -- Battery10/LConn2
  Series RLC Load/LConn1 -- Battery9/LConn2 -- Voltage Measurement/LConn2
  Series RLC Load/RConn1 -- Battery10/LConn1 -- Voltage Measurement/LConn1

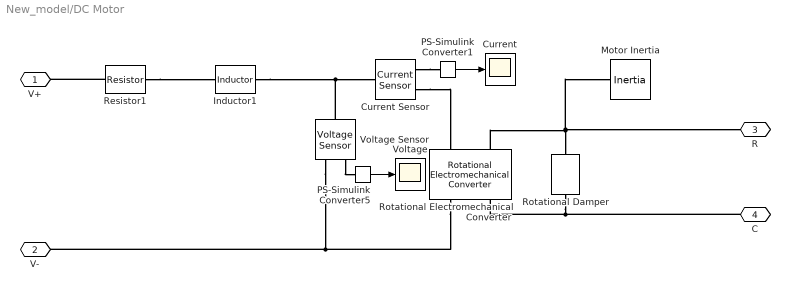
== system New_model/DC Motor ==
  " Motor Inertia" : fl_lib/Mechanical/Rotational Elements/Inertia  inertia=5.48e-5 kg*m^2  num_ports=foundation.enum.numPorts2.one  w_specify=off  w_priority=High  w=0 rad/s  w_nominal_specify=off  w_nominal_unit=rad/s  w_nominal_value=1  t_specify=off  t_priority=None  t=0 N*m  t_nominal_specify=off  t_nominal_unit=N*m  t_nominal_value=1
  Current : Scope
  Current Sensor : fl_lib/Electrical/Electrical Sensors/Current Sensor
  Inductor1 : fl_lib/Electrical/Electrical Elements/Inductor  l=0.072e-3 H  r=0 Ohm  g=1e-9 1/Ohm  i_specify=off  i_priority=None  i=0 A  i_nominal_specify=off  i_nominal_unit=A  i_nominal_value=1  v_specify=off  v_priority=None  v=0 V  v_nominal_specify=off  v_nominal_unit=V  v_nominal_value=1  i_L_specify=off  i_L_priority=High  i_L=0 A  i_L_nominal_specify=off  i_L_nominal_unit=A  i_L_nominal_value=1
  PS-Simulink Converter1 : nesl_utility/PS-Simulink Converter  PhysicalDomain=network_engine_domain  SubClassName=ps_output  LeftPortType=input  RightPortType=output  PseudoPeriodic=off  Frequencies=[]  Unit=inherit  AffineConversion=off
      settings: SourceProductBaseCode=PW,SS
  PS-Simulink Converter5 : nesl_utility/PS-Simulink Converter  PhysicalDomain=network_engine_domain  SubClassName=ps_output  LeftPortType=input  RightPortType=output  PseudoPeriodic=off  Frequencies=[]  Unit=inherit  AffineConversion=off
      settings: SourceProductBaseCode=PW,SS
  Resistor1 : fl_lib/Electrical/Electrical Elements/Resistor  R=0.103 Ohm  i_specify=off  i_priority=None  i=0 A  i_nominal_specify=off  i_nominal_unit=A  i_nominal_value=1  v_specify=off  v_priority=None  v=0 V  v_nominal_specify=off  v_nominal_unit=V  v_nominal_value=1
  Rotational Electromechanical Converter : fl_lib/Electrical/Electrical Elements/Rotational Electromechanical Converter  K=0.0385 V/(rad/s)  i_specify=off  i_priority=None  i=0 A  i_nominal_specify=off  i_nominal_unit=A  i_nominal_value=1  v_specify=off  v_priority=None  v=0 V  v_nominal_specify=off  v_nominal_unit=V  v_nominal_value=1  t_specify=off  t_priority=None  t=0 N*m  t_nominal_specify=off  t_nominal_unit=N*m  t_nominal_value=1  w_specify=off  w_priority=None  w=0 rad/s  w_nominal_specify=off  w_nominal_unit=rad/s  w_nominal_value=1
  Rotational Damper : fl_lib/Mechanical/Rotational Elements/Rotational Damper  D=2.458e-4 N*m/(rad/s)  w_specify=off  w_priority=None  w=0 rad/s  w_nominal_specify=off  w_nominal_unit=rad/s  w_nominal_value=1  t_specify=off  t_priority=None  t=0 N*m  t_nominal_specify=off  t_nominal_unit=N*m  t_nominal_value=1
  Voltage : Scope
  Voltage Sensor : fl_lib/Electrical/Electrical Sensors/Voltage Sensor
  V+ : PMIOPort  Side=Left
  V- : PMIOPort  Port=2  Side=Left
  R : PMIOPort  Port=3  Side=Right
  C : PMIOPort  Port=4  Side=Right
  wires:
  PS-Simulink Converter5/1 -> Voltage/1
  PS-Simulink Converter1/1 -> Current/1
  connections:
  Rotational Electromechanical Converter/LConn2 -- " Motor Inertia"/LConn1 -- R/RConn1 -- Rotational Damper/LConn1
  Resistor1/LConn1 -- V+/RConn1
  Rotational Damper/RConn1 -- C/RConn1 -- Rotational Electromechanical Converter/RConn2
  Rotational Electromechanical Converter/RConn1 -- Voltage Sensor/RConn2 -- V-/RConn1
  Voltage Sensor/RConn1 -- PS-Simulink Converter5/LConn1
  Current Sensor/RConn2 -- Rotational Electromechanical Converter/LConn1
  Current Sensor/RConn1 -- PS-Simulink Converter1/LConn1
  Resistor1/RConn1 -- Inductor1/LConn1
  Inductor1/RConn1 -- Voltage Sensor/LConn1 -- Current Sensor/LConn1

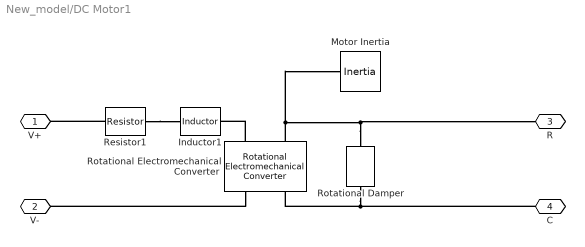
== system New_model/DC Motor1 ==
  " Motor Inertia" : fl_lib/Mechanical/Rotational Elements/Inertia  inertia=0.01 kg*m^2  num_ports=foundation.enum.numPorts2.one  w_specify=off  w_priority=High  w=0 rad/s  w_nominal_specify=off  w_nominal_unit=rad/s  w_nominal_value=1  t_specify=off  t_priority=None  t=0 N*m  t_nominal_specify=off  t_nominal_unit=N*m  t_nominal_value=1
  Inductor1 : fl_lib/Electrical/Electrical Elements/Inductor  l=1e-6 H  r=0 Ohm  g=1e-9 1/Ohm  i_specify=off  i_priority=None  i=0 A  i_nominal_specify=off  i_nominal_unit=A  i_nominal_value=1  v_specify=off  v_priority=None  v=0 V  v_nominal_specify=off  v_nominal_unit=V  v_nominal_value=1  i_L_specify=off  i_L_priority=High  i_L=0 A  i_L_nominal_specify=off  i_L_nominal_unit=A  i_L_nominal_value=1
  Resistor1 : fl_lib/Electrical/Electrical Elements/Resistor  R=1 Ohm  i_specify=off  i_priority=None  i=0 A  i_nominal_specify=off  i_nominal_unit=A  i_nominal_value=1  v_specify=off  v_priority=None  v=0 V  v_nominal_specify=off  v_nominal_unit=V  v_nominal_value=1
  Rotational Electromechanical Converter : fl_lib/Electrical/Electrical Elements/Rotational Electromechanical Converter  K=0.1 V/(rad/s)  i_specify=off  i_priority=None  i=0 A  i_nominal_specify=off  i_nominal_unit=A  i_nominal_value=1  v_specify=off  v_priority=None  v=0 V  v_nominal_specify=off  v_nominal_unit=V  v_nominal_value=1  t_specify=off  t_priority=None  t=0 N*m  t_nominal_specify=off  t_nominal_unit=N*m  t_nominal_value=1  w_specify=off  w_priority=None  w=0 rad/s  w_nominal_specify=off  w_nominal_unit=rad/s  w_nominal_value=1
  Rotational Damper : fl_lib/Mechanical/Rotational Elements/Rotational Damper  D=0.001 N*m/(rad/s)  w_specify=off  w_priority=None  w=0 rad/s  w_nominal_specify=off  w_nominal_unit=rad/s  w_nominal_value=1  t_specify=off  t_priority=None  t=0 N*m  t_nominal_specify=off  t_nominal_unit=N*m  t_nominal_value=1
  V+ : PMIOPort  Side=Left
  V- : PMIOPort  Port=2  Side=Left
  R : PMIOPort  Port=3  Side=Right
  C : PMIOPort  Port=4  Side=Right
  connections:
  Rotational Damper/LConn1 -- " Motor Inertia"/LConn1 -- Rotational Electromechanical Converter/LConn2 -- R/RConn1
  Resistor1/RConn1 -- Inductor1/LConn1
  Resistor1/LConn1 -- V+/RConn1
  Rotational Electromechanical Converter/RConn2 -- Rotational Damper/RConn1 -- C/RConn1
  Rotational Electromechanical Converter/RConn1 -- V-/RConn1
  Rotational Electromechanical Converter/LConn1 -- Inductor1/RConn1

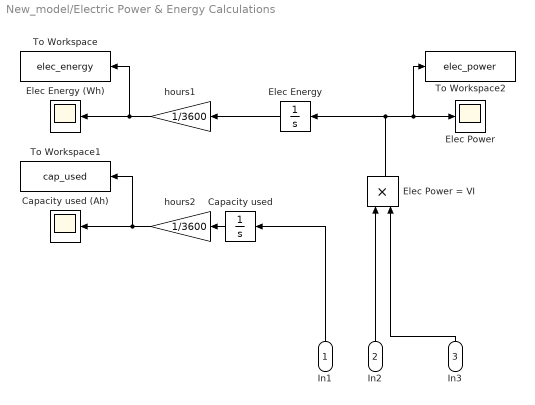
== system New_model/Electric Power & Energy Calculations ==
  In1 : Inport
  In2 : Inport  Port=2
  In3 : Inport  Port=3
  Capacity used : Integrator
  Capacity used (Ah) : Scope
  Elec Energy : Integrator
  Elec Energy (Wh) : Scope
  Elec Power : Scope
  Elec Power = VI : Product
  To Workspace : ToWorkspace  VariableName=elec_energy  SaveFormat=Timeseries  SampleTime=-1
  To Workspace1 : ToWorkspace  VariableName=cap_used  SaveFormat=Timeseries  SampleTime=-1
  To Workspace2 : ToWorkspace  VariableName=elec_power  SaveFormat=Timeseries  SampleTime=-1
  hours1 : Gain  Gain=1/3600
  hours2 : Gain  Gain=1/3600
  wires:
  hours1/1 -> To Workspace/1, Elec Energy (Wh)/1
  In2/1 -> Elec Power = VI/1
  hours2/1 -> Capacity used (Ah)/1, To Workspace1/1
  Elec Power = VI/1 -> Elec Energy/1, To Workspace2/1, Elec Power/1
  In1/1 -> Capacity used/1
  Elec Energy/1 -> hours1/1
  Capacity used/1 -> hours2/1
  In3/1 -> Elec Power = VI/2

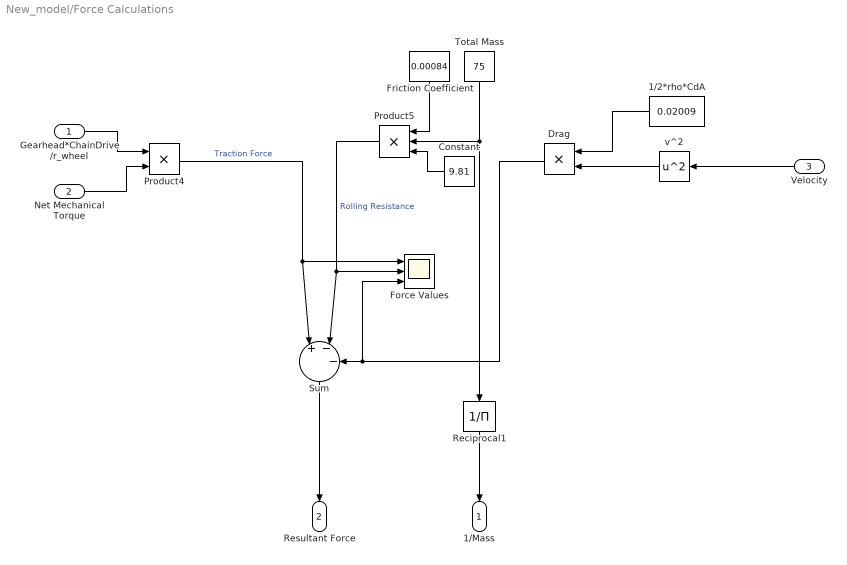
== system New_model/Force Calculations ==
  Gearhead*ChainDrive/r_wheel : Inport
  Net Mechanical Torque : Inport  Port=2
  Velocity : Inport  Port=3
  1/2*rho*CdA : Constant  Value=0.02009
  Constant : Constant  Value=9.81
  Drag : Product
  Force Values : Scope  NumInputPorts=3
  Friction Coefficient : Constant  Value=0.00084
  Product4 : Product
  Product5 : Product  Inputs=3
  Reciprocal1 : Product  Inputs=/
  Sum : Sum  Inputs=|+--
  Total Mass : Constant  Value=75
  v^2 : Math  Operator=square  SaturateOnIntegerOverflow=on
  1/Mass : Outport
  Resultant Force : Outport  Port=2
  wires:
  Product4/1 -> Force Values/1, Sum/1  "Traction Force"
  Total Mass/1 -> Reciprocal1/1, Product5/2
  v^2/1 -> Drag/2
  Constant/1 -> Product5/3
  Product5/1 -> Force Values/2, Sum/2  "Rolling Resistance"
  Drag/1 -> Force Values/3, Sum/3
  1/2*rho*CdA/1 -> Drag/1
  Friction Coefficient/1 -> Product5/1
  Velocity/1 -> v^2/1
  Net Mechanical Torque/1 -> Product4/2
  Gearhead*ChainDrive/r_wheel/1 -> Product4/1
  Reciprocal1/1 -> 1/Mass/1
  Sum/1 -> Resultant Force/1

== matlab function New_model/Throttle & Voltage Control ==
  data: vol_input output; time input
function vol_input = throttle(time)

% if time == 0
%     velocity = 0;
% end
V_control = 24;

if time == 0
    vol_input = 0.5*V_control;
elseif time > 0 && time <= 20 
    vol_input = 0.5*V_control + time*(0.5*V_control)/20;
else
    vol_input = 24;
end

if time >= 60
    vol_input = 5.415;
%     vol_input = 6.3;
end


if vol_input > V_control
    vol_input = V_control;
end


    
end
